simulink model "CAVE_MachE_driver_test"  (R2024a)
settings: configuration reference "ConfigSetDesktopFixedStep" (kept outside this file)
PreLoadFcn:
  | VSS_BICYCLE=Simulink.Variant('Dual=0');
  | VSS_DUAL=Simulink.Variant('Dual=1');
  | Dual=1;
  | load('DriveCycle2.mat')
PostLoadFcn:
  | if any(exist('dsrtsu_mdlpostloadfcn', 'file') ~= 0), dsrtsu_mdlpostloadfcn('Execute', bdroot); end
InitFcn:
  | , if any(exist('rtifpga_mdlclblib', 'file') ~= 0), rtifpga_mdlclblib('Init', bdroot); end,
  | , if any(exist('dsmpb_private', 'file') ~= 0), dsmpb_private('dsmpb_mdlclblib', 'Init', bdroot); end,
  | load('DriveCycle2.mat')
model workspace (MAT data in the model file):
  Gas = 0.383333333333
values from neighbouring files (symbols this model uses):
  CoastDown =     [Run_Simulink.mat]
  limitedMCT =     [Run_Simulink.mat]
  MCT =     [Run_Simulink.mat]
  optimized_speed = [6.8451519807e-19 6.71455685751e-19 6.61817305122e-19 6.79712455505e-19 6.66916107161e-19 6.93956205717e-19 6.71488581248e-19 6.61948887111e-19 6.81653289829e-19 6.68560882013e-19 6.9214695338e-19 6.73330729082e-19 ... (16417 elements, 16417x1)]    [OptimizedSpeed.mat]
  optimized_speed_time = [0 0.1 0.2 0.3 0.4 0.5 0.6 0.7 0.8 0.9 1 1.1 ... (16417 elements, 16417x1)]    [OptimizedSpeed.mat]
  pMCT =     [Run_Simulink.mat]
  RealSimPara =     [Run_Simulink.mat]
  Ref_speed = [13 13.007895099 13.015778396 13.023649891 13.031509584 13.039357475 13.047193564 13.055017851 13.062830336 13.070631019 13.0784199 13.086196979 ... (2669 elements, 2669x1)]    [Ref_speed_and_time.mat]
  Ref_time = [0 0.01 0.02 0.03 0.04 0.05 0.06 0.07 0.08 0.09 0.1 0.11 ... (2669 elements, 2669x1)]    [Ref_speed_and_time.mat]
  US06 =     [Run_Simulink.mat]
undefined symbols (not defined in the file or in its folder): AccelCmd, ActTqLF_Nm_, ActTqLR_Nm_, ActTqRF_Nm_, ActTqRR_Nm_, BattChargeLimitMaxPwr, BattChargeLimitSocBpts, BattChargeLimitTbl, BattChrgCapcty, BattDischargeLimitSocBpts, BattDischargeLimitTbl, BattDischargeMaxPwr, BattNumCellsParallel, BattNumCellsSeries, BattOpenVoltCapBpts, BattOpenVoltTbl, BattResistSocBpts, BattResistTbl, BattResistTempBpts, BrakeMaxPrs, BrakeMaxTrq, ChassisDistCg2FrontAxle, ChassisDistCg2RearAxle, ChassisVehMass, CltchCmd, DecelCmd, DiffRatio, DiscIntNeverNeededParam, EnvGravCnst, EnvPrs, EnvTemp, FuelSpecificGrav, GearCmd, h, InitStates, lgSw, MtrEffSpdBpts, MtrEffTbl, MtrEffTrqBpts, MtrPwrMax, MtrTrqMax, ResultsDrivingTests, SteeringCmd, SupvsryCtrlRegenBrkCutOffTbl, SupvsryCtrlRegenSpdBpts, TestScnrioCycleNum, VEH
libraries: simulink x122, VSIGenLib x122, etargetslib x75, dsmpblib x55, vehdynlibtire x24, autolibshared x22, CarMaker4SL x20, vehdynlibsuspension x14, vehdynlibtirecommon x14, autolibutils x10, VsrLibWheel x8, autolibpowerinfoutils x6
(part 12 of 32)

== system CAVE_MachE_driver_test/Vehicle Under Test3/Vehicle/Battery/Battery/Lithium Ion Battery Pack1 ==
  note: Info
  BattCurr : Inport  Unit=A
  BattTemp : Inport  Port=2  Unit=K
  Datasheet Battery Internal : Subsystem  AncestorBlock=autolibbatterycommon/Datasheet Battery Internal
  Info Bus : autolibbatterycommon/Info  RefBlkName='autolibdatasheetbattery/Datasheet Battery'
  Output Passthrough : autolibbatterycommon/Output Passthrough  SystemSampleTime=-1  VariantActivationTime=update diagram  AllowFlexibleInterface=on  Latency=0  AutoFrameSizeCalculation=off
  Info : Outport  VectorParamsAs1DForOutWhenUnconnected=off
  BattVolt : Outport  Port=2  Unit=V  VectorParamsAs1DForOutWhenUnconnected=off
  wires:
  [BattPwrLoss] -> Info Bus/5
  Output Passthrough/1 -> BattVolt/1, [BattVolt]
  [BattVolt] -> Info Bus/4
  Datasheet Battery Internal/1(LdCurrFeed) -> [LdCurrFeed]
  [LdCurrFeed] -> Info Bus/3
  Datasheet Battery Internal/5(BattPwrLoss) -> [BattPwrLoss]
  Datasheet Battery Internal/2(OutVoltUnfilt) -> Output Passthrough/1
  Datasheet Battery Internal/3(LdAmpHr) -> [LdAmpHr]
  Datasheet Battery Internal/4(BattSoc) -> [BattSoc]
  BattTemp/1 -> Datasheet Battery Internal/2(BattTemp)
  BattCurr/1 -> Datasheet Battery Internal/1(BattCurr)
  Info Bus/1 -> Info/1
  [BattSoc] -> Info Bus/2
  [LdAmpHr] -> Info Bus/1

== system CAVE_MachE_driver_test/Vehicle Under Test3/Vehicle/Driver and Drive Cycle/Driver and PI with FF Control/Speed controller set ==
  RefSpd [km/hr] : Inport
  VehSpd : Inport  Port=2
  Control selection : Constant
  In-house CAVE : Subsystem  VariantControl=varaint1
  Multiport Switch1 : MultiPortSwitch  SaturateOnIntegerOverflow=off  InputSameDT=off
  Multiport Switch2 : MultiPortSwitch  SaturateOnIntegerOverflow=off  InputSameDT=off
  Multiport Switch3 : MultiPortSwitch  SaturateOnIntegerOverflow=off  InputSameDT=off
  PIF : Subsystem  VariantControl=varaint2
  Predictive : Subsystem  VariantControl=varaint3
  Scope : Scope  NumInputPorts=2
  Speed tracking controller : Subsystem  Commented=on  Variant=on  VariantControlMode=label  VariantControl=Variant1  LabelModeActiveChoice=varaint1  PropagateVariantConditions=on
  Out1 : Outport
  Out2 : Outport  Port=2
  Out3 : Outport  Port=3
  wires:
  Control selection/1 -> Multiport Switch3/1, Multiport Switch2/1, Multiport Switch1/1
  RefSpd [km/hr]/1 -> Scope/1, In-house CAVE/1(RefSpd [km/hr]), Predictive/1(RefSpd [km/hr]), PIF/1(RefSpd [km/hr])
  In-house CAVE/1(AccelPedalCmd) -> Multiport Switch1/2
  PIF/1(AccelPedalCmd) -> Multiport Switch1/3
  Predictive/1(AccelPedalCmd) -> Multiport Switch1/4
  In-house CAVE/2(BrakePedalCmd) -> Multiport Switch2/2
  PIF/2(BrakePedalCmd) -> Multiport Switch2/3
  Predictive/2(BrakePedalCmd) -> Multiport Switch2/4
  In-house CAVE/3(Out3) -> Multiport Switch3/2
  PIF/3(Out3) -> Multiport Switch3/3
  Predictive/3(Out3) -> Multiport Switch3/4
  Multiport Switch3/1 -> Out3/1  "BrakeSwitch"
  Multiport Switch2/1 -> Out2/1  "BrakePedalCmd"
  Multiport Switch1/1 -> Out1/1  "AccelPedalCmd"
  VehSpd/1 -> Scope/2, In-house CAVE/2(In2), PIF/2(In2), Predictive/2(In2)

== system CAVE_MachE_driver_test/Vehicle Under Test3/Vehicle/Front Wheel Drive/Ideal Diff/Power Bus ==
  DriveshftTrq : Inport
  Speed : Inport  Port=2
  Bus Creator : BusCreator  Inputs=1
  Bus Creator5 : BusCreator  Inputs=2
  Bus Creator6 : BusCreator  Inputs=3
  Bus Creator7 : BusCreator  Inputs=1
  Constant : Constant  Value=0
  Constant1 : Constant  Value=0
  Constant2 : Constant  Value=0
  Demux : Demux  Outputs=3
  Power Accounting Bus Creator : autolibpowerinfoutils/Power Accounting Bus Creator  AssctBlkSelPopup=Parent reference block  RefBlkName='autolibshareddiff/Open Differential'  PwrTrnsfrdCheckBox=on  PwrNotTrnsfrdCheckBox=on  PwrStoredCheckBox=on  aMode=aMode
  Signal Specification5 : SignalSpecification  Unit=W
  Transferred Power : Product
  Vector Concatenate : Concatenate  NumInputs=3
  PwrInfo : Outport
  wires:
  Bus Creator/1 -> Power Accounting Bus Creator/1
  Power Accounting Bus Creator/1 -> PwrInfo/1  "PwrInfo"
  Bus Creator5/1 -> Power Accounting Bus Creator/2
  Bus Creator6/1 -> Bus Creator/1  "PwrTrnsfrd"
  Transferred Power/1 -> Signal Specification5/1
  Signal Specification5/1 -> Vector Concatenate/3, Vector Concatenate/2, Vector Concatenate/1  "PwrDriveshft"
  Constant/1 -> Bus Creator5/1  "PwrMechLoss"
  Demux/3 -> Bus Creator6/3  "PwrAxl2"
  DriveshftTrq/1 -> Transferred Power/1
  Bus Creator7/1 -> Power Accounting Bus Creator/3
  Demux/2 -> Bus Creator6/2  "PwrAxl1"
  Demux/1 -> Bus Creator6/1  "PwrDriveshft"
  Speed/1 -> Transferred Power/2
  Vector Concatenate/1 -> Demux/1
  Constant1/1 -> Bus Creator5/2  "PwrDampLoss"
  Constant2/1 -> Bus Creator7/1  "PwrStoredShft"

== system CAVE_MachE_driver_test/Vehicle Under Test3/Vehicle/Front Wheel Drive/Ideal Diff AWD/Power Bus ==
  DriveshftTrq : Inport
  Speed : Inport  Port=2
  Bus Creator : BusCreator  Inputs=1
  Bus Creator5 : BusCreator  Inputs=2
  Bus Creator6 : BusCreator  Inputs=3
  Bus Creator7 : BusCreator  Inputs=1
  Constant : Constant  Value=0
  Constant1 : Constant  Value=0
  Constant2 : Constant  Value=0
  Demux : Demux  Outputs=3
  Power Accounting Bus Creator : autolibpowerinfoutils/Power Accounting Bus Creator  AssctBlkSelPopup=Parent reference block  RefBlkName='autolibshareddiff/Open Differential'  PwrTrnsfrdCheckBox=on  PwrNotTrnsfrdCheckBox=on  PwrStoredCheckBox=on  aMode=aMode
  Signal Specification5 : SignalSpecification  Unit=W
  Transferred Power : Product
  Vector Concatenate : Concatenate  NumInputs=3
  PwrInfo : Outport
  wires:
  Bus Creator/1 -> Power Accounting Bus Creator/1
  Power Accounting Bus Creator/1 -> PwrInfo/1  "PwrInfo"
  Bus Creator5/1 -> Power Accounting Bus Creator/2
  Bus Creator6/1 -> Bus Creator/1  "PwrTrnsfrd"
  Transferred Power/1 -> Signal Specification5/1
  Signal Specification5/1 -> Vector Concatenate/3, Vector Concatenate/2, Vector Concatenate/1  "PwrDriveshft"
  Constant/1 -> Bus Creator5/1  "PwrMechLoss"
  Demux/3 -> Bus Creator6/3  "PwrAxl2"
  DriveshftTrq/1 -> Transferred Power/1
  Bus Creator7/1 -> Power Accounting Bus Creator/3
  Demux/2 -> Bus Creator6/2  "PwrAxl1"
  Demux/1 -> Bus Creator6/1  "PwrDriveshft"
  Speed/1 -> Transferred Power/2
  Vector Concatenate/1 -> Demux/1
  Constant1/1 -> Bus Creator5/2  "PwrDampLoss"
  Constant2/1 -> Bus Creator7/1  "PwrStoredShft"

== system CAVE_MachE_driver_test/Vehicle Under Test3/Vehicle/Front Wheel Drive/Real Diff/Power Bus ==
  DriveshftTrq : Inport
  Speed : Inport  Port=2
  Bus Creator : BusCreator  Inputs=1
  Bus Creator5 : BusCreator  Inputs=2
  Bus Creator6 : BusCreator  Inputs=3
  Bus Creator7 : BusCreator  Inputs=1
  Constant : Constant  Value=0
  Constant1 : Constant  Value=0
  Constant2 : Constant  Value=0
  Demux : Demux  Outputs=3
  Power Accounting Bus Creator : autolibpowerinfoutils/Power Accounting Bus Creator  AssctBlkSelPopup=Parent reference block  RefBlkName='autolibshareddiff/Open Differential'  PwrTrnsfrdCheckBox=on  PwrNotTrnsfrdCheckBox=on  PwrStoredCheckBox=on  aMode=aMode
  Signal Specification5 : SignalSpecification  Unit=W
  Transferred Power : Product
  Vector Concatenate : Concatenate  NumInputs=3
  PwrInfo : Outport
  wires:
  Bus Creator/1 -> Power Accounting Bus Creator/1
  Power Accounting Bus Creator/1 -> PwrInfo/1  "PwrInfo"
  Bus Creator5/1 -> Power Accounting Bus Creator/2
  Bus Creator6/1 -> Bus Creator/1  "PwrTrnsfrd"
  Transferred Power/1 -> Signal Specification5/1
  Signal Specification5/1 -> Vector Concatenate/3, Vector Concatenate/2, Vector Concatenate/1  "PwrDriveshft"
  Constant/1 -> Bus Creator5/1  "PwrMechLoss"
  Demux/3 -> Bus Creator6/3  "PwrAxl2"
  DriveshftTrq/1 -> Transferred Power/1
  Bus Creator7/1 -> Power Accounting Bus Creator/3
  Demux/2 -> Bus Creator6/2  "PwrAxl1"
  Demux/1 -> Bus Creator6/1  "PwrDriveshft"
  Speed/1 -> Transferred Power/2
  Vector Concatenate/1 -> Demux/1
  Constant1/1 -> Bus Creator5/2  "PwrDampLoss"
  Constant2/1 -> Bus Creator7/1  "PwrStoredShft"

== system CAVE_MachE_driver_test/Vehicle Under Test3/Vehicle/Powertrain Supervisory Controller /Engine Torque Command/Accel Pedal to Traction Wheel Torque Request1 ==
  note: Convert Accelerator Pedal Position to Torque Command
      | using Motor Torque Speed Curve
  AccelPdl : Inport
  MotSpd : Inport  Port=2
  Max Motor Torque : Subsystem
  Product1 : Product
  TrqCmd : Outport  VectorParamsAs1DForOutWhenUnconnected=off
  wires:
  Max Motor Torque/1(MtrTrqMax) -> Product1/2
  MotSpd/1 -> Max Motor Torque/1(MtrSpd)
  AccelPdl/1 -> Product1/1
  Product1/1 -> TrqCmd/1

== system CAVE_MachE_driver_test/Vehicle Under Test3/Vehicle/Powertrain Supervisory Controller /Engine Torque Command/Battery Management System ==
  note: Behaviorial BMS System. Limits battery charge / discharge power based on SOC.
      |
      | Charge/Discharge Limits and curves can be adjusted if using a larger battery pack
      | or motor power is changed.
  SOC : Inport
  ChrgLmt : Lookup_n-D  NumberOfTableDimensions=1  BreakpointsForDimension1=BattChargeLimitSocBpts  Table=BattChargeLimitTbl  ExtrapMethod=Clip  UseLastTableValue=on  InternalRulePriority=Speed  RndMeth=Simplest
  DischrgLmt : Lookup_n-D  NumberOfTableDimensions=1  BreakpointsForDimension1=BattDischargeLimitSocBpts  Table=BattDischargeLimitTbl  ExtrapMethod=Clip  UseLastTableValue=on  InternalRulePriority=Speed  RndMeth=Simplest
  MaxChrg : Constant  Value=BattChargeLimitMaxPwr
  MaxDischrg : Constant  Value=BattDischargeMaxPwr
  Product : Product
  Product1 : Product
  BattPwrDischrgLmt : Outport  VectorParamsAs1DForOutWhenUnconnected=off
  BattPwrChrgLmt : Outport  Port=2  VectorParamsAs1DForOutWhenUnconnected=off
  wires:
  DischrgLmt/1 -> Product/1
  ChrgLmt/1 -> Product1/1
  Product1/1 -> BattPwrChrgLmt/1
  Product/1 -> BattPwrDischrgLmt/1
  MaxDischrg/1 -> Product/2
  MaxChrg/1 -> Product1/2
  SOC/1 -> ChrgLmt/1, DischrgLmt/1

== system CAVE_MachE_driver_test/Vehicle Under Test3/Vehicle/Powertrain Supervisory Controller /Engine Torque Command/Motor Torque Arbitration and Power Management ==
  MotTrqCmdTrac : Inport
  AccelPdl : Inport  Port=2
  BattPwrDisChrgLmt : Inport  Port=3
  "BattPwrChrgLmt " : Inport  Port=4
  MotSpd : Inport  Port=5
  MotTrqCmdRegen : Inport  Port=6
  Accel Decel Switch : Switch  Criteria=u2 > Threshold  SaturateOnIntegerOverflow=off  InputSameDT=off
  Compare To Constant : simulink/Logic and Bit Operations/Compare To Constant  relop=>  const=0  OutDataTypeStr=boolean
  Power Management : Subsystem
  MotTrqCmdFinal : Outport  VectorParamsAs1DForOutWhenUnconnected=off
  wires:
  Compare To Constant/1 -> Accel Decel Switch/2
  MotSpd/1 -> Power Management/3(MotSpd)
  "BattPwrChrgLmt "/1 -> Power Management/2(BattPwrChrgLmt)
  BattPwrDisChrgLmt/1 -> Power Management/1(BattPwrDischrgLmt)
  Accel Decel Switch/1 -> Power Management/4(MotTrqCmd)
  Power Management/1(MotTrqCmdFinal) -> MotTrqCmdFinal/1
  MotTrqCmdTrac/1 -> Accel Decel Switch/1
  MotTrqCmdRegen/1 -> Accel Decel Switch/3
  AccelPdl/1 -> Compare To Constant/1

== system CAVE_MachE_driver_test/Vehicle Under Test3/Vehicle/Powertrain Supervisory Controller /Engine Torque Command/Series Regen Braking ==
  note: These are all torque on wheels, which is DiffRatio*torque on motor
  note: - Total brake torque request based on brake pressure and parameters of disc brakes
      | - Use as much regenerative motor braking as possible
      | - Any braking torque request that cannot be provided by the motor, will be provided by the friction brakes
  BattSoc : Inport
  VehSpd : Inport  Port=2
  MotSpd : Inport  Port=3
  "DecelCmd " : Inport  Port=4
  ChrgLmt : Lookup_n-D  NumberOfTableDimensions=1  BreakpointsForDimension1=BattChargeLimitSocBpts  Table=BattChargeLimitTbl  ExtrapMethod=Clip  UseLastTableValue=on  InternalRulePriority=Speed  RndMeth=Simplest
  Gain : Gain  Gain=-1
  Gain1 : Gain  Gain=BrakeMaxTrq
  Gain2 : Gain  Gain=1/BrakeMaxTrq
  Max Motor Torque : LibPtSupervisoryCtrl/Powertrain Supervisory Controller /Engine Torque Command/Accel Pedal to Traction Wheel Torque Request/Max Motor Torque  SystemSampleTime=-1  VariantActivationTime=update diagram  AllowFlexibleInterface=on  Latency=0  AutoFrameSizeCalculation=off
  MinMax : MinMax  Inputs=2
  MotTrqReflectedToWheels : Gain  Gain=DiffRatio
  Product1 : Product
  Product3 : Product
  RegenBrakingCutoff : Lookup_n-D  NumberOfTableDimensions=1  BreakpointsForDimension1=SupvsryCtrlRegenSpdBpts  Table=SupvsryCtrlRegenBrkCutOffTbl  ExtrapMethod=Clip  UseLastTableValue=on  InternalRulePriority=Speed  RndMeth=Simplest
  Saturation : Saturate  UpperLimit=1  LowerLimit=0
  Saturation1 : Saturate  UpperLimit=1  LowerLimit=0
  Subtract : Sum  Inputs=+-
  WhlTrqReflectedToMot : Gain  Gain=1/DiffRatio
  " MotTrqCmdRegen" : Outport  VectorParamsAs1DForOutWhenUnconnected=off
  " BrkCmd" : Outport  Port=2  VectorParamsAs1DForOutWhenUnconnected=off
  wires:
  Gain2/1 -> Saturation1/1  "BrkTrqReqTotal"
  Subtract/1 -> Gain2/1
  Saturation/1 -> Gain1/1
  "DecelCmd "/1 -> Saturation/1  "BrkPrsReq"
  Gain/1 -> " MotTrqCmdRegen"/1  "MotTrqCmdRegen"
  WhlTrqReflectedToMot/1 -> Gain/1
  MotTrqReflectedToWheels/1 -> MinMax/2  "MotTrqMaxWhls"
  MotSpd/1 -> Max Motor Torque/1
  BattSoc/1 -> ChrgLmt/1
  Product1/1 -> Product3/2  "RegenFactor"
  RegenBrakingCutoff/1 -> Product1/1
  VehSpd/1 -> RegenBrakingCutoff/1
  ChrgLmt/1 -> Product1/2
  MinMax/1 -> Product3/1  "min"
  Max Motor Torque/1 -> MotTrqReflectedToWheels/1  "MotTrqMax"
  Saturation1/1 -> " BrkCmd"/1
  Product3/1 -> Subtract/2, WhlTrqReflectedToMot/1  "MotTrqRegenWhl"
  Gain1/1 -> MinMax/1, Subtract/1  "BrkTrqReqTotal"

== system CAVE_MachE_driver_test/Vehicle Under Test3/Vehicle/Rototest and ORNL Interface/From Rototest/RotoTestEthRX ==
  Input : Inport
  Depacker : Subsystem
  Floater{,1..15} (16 alike) : VSIGenLib/Floater  SystemSampleTime=-1  VariantActivationTime=update diagram  AllowFlexibleInterface=on  Latency=0  AutoFrameSizeCalculation=off
  Header : VSIGenLib/Header  not=''
  Selector1 : Selector  IndexMode=Zero-based  InputPortWidth=96  IndexOptions=Index vector (dialog)  Indices=[3 2]  OutputSizes=1
  Selector10 : Selector  IndexMode=Zero-based  InputPortWidth=96  IndexOptions=Index vector (dialog)  Indices=[35 34 33 32]  OutputSizes=1
  Selector11 : Selector  IndexMode=Zero-based  InputPortWidth=96  IndexOptions=Index vector (dialog)  Indices=[39 38 37 36]  OutputSizes=1
  Selector12 : Selector  IndexMode=Zero-based  InputPortWidth=96  IndexOptions=Index vector (dialog)  Indices=[43 42 41 40]  OutputSizes=1
  Selector13 : Selector  IndexMode=Zero-based  InputPortWidth=96  IndexOptions=Index vector (dialog)  Indices=[47 46 45 44]  OutputSizes=1
  Selector14 : Selector  IndexMode=Zero-based  InputPortWidth=96  IndexOptions=Index vector (dialog)  Indices=[51 50 49 48]  OutputSizes=1
  Selector15 : Selector  IndexMode=Zero-based  InputPortWidth=96  IndexOptions=Index vector (dialog)  Indices=[55 54 53 52]  OutputSizes=1
  Selector16 : Selector  IndexMode=Zero-based  InputPortWidth=96  IndexOptions=Index vector (dialog)  Indices=[59 58 57 56]  OutputSizes=1
  Selector17 : Selector  IndexMode=Zero-based  InputPortWidth=96  IndexOptions=Index vector (dialog)  Indices=[63 62 61 60]  OutputSizes=1
  Selector18 : Selector  IndexMode=Zero-based  InputPortWidth=96  IndexOptions=Index vector (dialog)  Indices=[67 66 65 64]  OutputSizes=1
  Selector19 : Selector  IndexMode=Zero-based  InputPortWidth=96  IndexOptions=Index vector (dialog)  Indices=[71 70 69 68]  OutputSizes=1
  Selector2 : Selector  IndexMode=Zero-based  InputPortWidth=96  IndexOptions=Index vector (dialog)  Indices=[7 6 5 4]  OutputSizes=1
  Selector20 : Selector  IndexMode=Zero-based  InputPortWidth=96  IndexOptions=Index vector (dialog)  Indices=[75 74 73 72]  OutputSizes=1
  Selector21 : Selector  IndexMode=Zero-based  InputPortWidth=96  IndexOptions=Index vector (dialog)  Indices=[79 78 77 76]  OutputSizes=1
  Selector22 : Selector  IndexMode=Zero-based  InputPortWidth=96  IndexOptions=Index vector (dialog)  Indices=[83 82 81 80]  OutputSizes=1
  Selector23 : Selector  IndexMode=Zero-based  InputPortWidth=96  IndexOptions=Index vector (dialog)  Indices=[85 84]  OutputSizes=1
  Selector24 : Selector  IndexMode=Zero-based  InputPortWidth=96  IndexOptions=Index vector (dialog)  Indices=[87 86]  OutputSizes=1
  Selector25 : Selector  IndexMode=Zero-based  InputPortWidth=96  IndexOptions=Index vector (dialog)  Indices=[89 88]  OutputSizes=1
  Selector26 : Selector  IndexMode=Zero-based  InputPortWidth=96  IndexOptions=Index vector (dialog)  Indices=[91 90]  OutputSizes=1
  Selector27 : Selector  IndexMode=Zero-based  InputPortWidth=96  IndexOptions=Index vector (dialog)  Indices=[93 92]  OutputSizes=1
  Selector28 : Selector  IndexMode=Zero-based  InputPortWidth=96  IndexOptions=Index vector (dialog)  Indices=[94]  OutputSizes=1
  Selector29 : Selector  IndexMode=Zero-based  InputPortWidth=96  IndexOptions=Index vector (dialog)  Indices=[95]  OutputSizes=1
  Selector3 : Selector  IndexMode=Zero-based  InputPortWidth=96  IndexOptions=Index vector (dialog)  Indices=[1 0]  OutputSizes=1
  Selector4 : Selector  IndexMode=Zero-based  InputPortWidth=96  IndexOptions=Index vector (dialog)  Indices=[11 10 9 8]  OutputSizes=1
  Selector5 : Selector  IndexMode=Zero-based  InputPortWidth=96  IndexOptions=Index vector (dialog)  Indices=[15 14 13 12]  OutputSizes=1
  Selector6 : Selector  IndexMode=Zero-based  InputPortWidth=96  IndexOptions=Index vector (dialog)  Indices=[19 18 17 16]  OutputSizes=1
  Selector7 : Selector  IndexMode=Zero-based  InputPortWidth=96  IndexOptions=Index vector (dialog)  Indices=[23 22 21 20]  OutputSizes=1
  Selector8 : Selector  IndexMode=Zero-based  InputPortWidth=96  IndexOptions=Index vector (dialog)  Indices=[27 26 25 24]  OutputSizes=1
  Selector9 : Selector  IndexMode=Zero-based  InputPortWidth=96  IndexOptions=Index vector (dialog)  Indices=[31 30 29 28]  OutputSizes=1
  Terminator{,1..2,7..8} (5 alike) : Terminator
  uint16 (unsigned 16){1..7} (7 alike) : etargetslib/Byte Unpack  dimensions={[1]}  datatypes={'uint16'}  byteAlign=1
  uint32 (unsigned 32){1..4} (4 alike) : etargetslib/Byte Unpack  dimensions={[1]}  datatypes={'uint32'}  byteAlign=1
  uint8 (unsigned 8)1 : etargetslib/Byte Unpack  dimensions={[1]}  datatypes={'uint8'}  byteAlign=1
  uint8 (unsigned 8)2 : etargetslib/Byte Unpack  dimensions={[1]}  datatypes={'uint8'}  byteAlign=1
  ID : Outport
  ProtocolVer : Outport  Port=2
  ActTqLF_Nm : Outport  Port=3
  ActSpLF_rpm : Outport  Port=4
  ActTempLF_C : Outport  Port=5
  ActTqRF_Nm_ : Outport  Port=6
  ActSpRF_rpm : Outport  Port=7
  ActTempRF_C : Outport  Port=8
  ActTqLR_Nm : Outport  Port=9
  ActSpLR_rpm : Outport  Port=10
  ActTempLR_C : Outport  Port=11
  ActTqRR_Nm : Outport  Port=12
  ActSpRR_rpm : Outport  Port=13
  ActTempRR_Nm : Outport  Port=14
  RefLF_Nm : Outport  Port=15
  RefRF_rpm : Outport  Port=16
  RefLR_Nm : Outport  Port=17
  RefRR_Nm : Outport  Port=18
  UnitsStatusLF : Outport  Port=19
  UnitsStatusRF : Outport  Port=20
  UnitsStatusLR : Outport  Port=21
  UnitsStatusRR : Outport  Port=22
  WatchdogCnt : Outport  Port=23
  FaultActive : Outport  Port=24
  WarningsActive : Outport  Port=25
  SpTqRR : Outport  Port=26
  SpTqLR : Outport  Port=27
  SpTqRF : Outport  Port=28
  SpTqLF : Outport  Port=29
  SystemActive : Outport  Port=30
  wires:
  Depacker/7(SystemActive) -> SystemActive/1
  Depacker/5(SpTqRF) -> SpTqRF/1
  Depacker/1(FaultActive) -> FaultActive/1
  Depacker/2(WarningsActive) -> WarningsActive/1
  Depacker/3(SpTqRR) -> SpTqRR/1
  Depacker/4(SpTqLR) -> SpTqLR/1
  Depacker/6(SpTqLF) -> SpTqLF/1
  Floater5/1 -> ActTempRF_C/1  "ActTempRF_C"
  uint32 (unsigned 32)2/1 -> Terminator1/1  "Reserved"
  Floater/1 -> ActSpLF_rpm/1  "ActSpLF_rpm"
  uint32 (unsigned 32)1/1 -> Terminator/1  "Reserved"
  uint16 (unsigned 16)1/1 -> ID/1  "ID"
  Floater15/1 -> RefRR_Nm/1  "RefRR_Nm"
  uint8 (unsigned 8)1/1 -> WatchdogCnt/1  "WatchdogCnt"
  Floater14/1 -> RefRF_rpm/1  "RefRF_rpm"
  uint16 (unsigned 16)5/1 -> UnitsStatusRF/1  "UnitsStatusRF"
  uint32 (unsigned 32)3/1 -> Terminator2/1  "Reserved"
  Floater9/1 -> ActSpRR_rpm/1  "ActSpRR_rpm"
  Floater1/1 -> ActTqLF_Nm/1  "ActTqLF_Nm_"
  Floater2/1 -> ActTempLF_C/1  "ActTempLF_C"
  Floater12/1 -> RefLF_Nm/1  "RefLF_Nm"
  Floater7/1 -> ActTqLR_Nm/1  "ActTqLR_Nm_"
  uint16 (unsigned 16)2/1 -> ProtocolVer/1  "ProtocolVer"
  Selector24/1 -> uint16 (unsigned 16)4/1
  Selector7/1 -> Floater4/1
  Selector8/1 -> Floater3/1
  uint16 (unsigned 16)7/1 -> UnitsStatusRR/1  "UnitsStatusRR"
  Selector22/1 -> Floater15/1
  Selector18/1 -> uint32 (unsigned 32)4/1
  Selector12/1 -> Floater6/1
  Selector23/1 -> uint16 (unsigned 16)3/1
  uint16 (unsigned 16)6/1 -> UnitsStatusLR/1  "UnitsStatusLR"
  Selector17/1 -> Floater11/1
  uint16 (unsigned 16)4/1 -> UnitsStatusLF/1  "UnitsStatusLF"
  Selector27/1 -> uint16 (unsigned 16)7/1
  Floater13/1 -> RefLR_Nm/1  "RefLR_Nm"
  Selector14/1 -> uint32 (unsigned 32)3/1
  Selector2/1 -> Floater1/1
  Selector13/1 -> Floater8/1
  Selector26/1 -> uint16 (unsigned 16)6/1
  Selector6/1 -> uint32 (unsigned 32)1/1
  uint16 (unsigned 16)3/1 -> Depacker/1(SysStsBits)  "SystemStatusBits"
  uint32 (unsigned 32)4/1 -> Terminator7/1  "Reserved"
  Floater3/1 -> ActSpRF_rpm/1  "ActSpRF_rpm"
  Selector25/1 -> uint16 (unsigned 16)5/1
  Floater4/1 -> ActTqRF_Nm_/1  "ActTqRF_Nm_"
  uint8 (unsigned 8)2/1 -> Terminator8/1  "Reserved"
  Floater11/1 -> ActTempRR_Nm/1  "ActTempRR_Nm"
  Floater6/1 -> ActSpLR_rpm/1  "ActSpLR_rpm"
  Selector20/1 -> Floater14/1
  Selector9/1 -> Floater5/1
  Selector5/1 -> Floater2/1
  Selector15/1 -> Floater10/1
  Selector16/1 -> Floater9/1
  Floater8/1 -> ActTempLR_C/1  "ActTempLR_C"
  Selector3/1 -> uint16 (unsigned 16)1/1
  Selector28/1 -> uint8 (unsigned 8)1/1
  Selector29/1 -> uint8 (unsigned 8)2/1
  Selector21/1 -> Floater13/1
  Input/1 -> Selector7/1, Selector8/1, Selector9/1, Selector10/1, Selector11/1, Selector12/1, Selector13/1, Selector17/1, Selector18/1, Selector19/1, Selector20/1, Selector21/1, Selector22/1, Selector23/1, Selector25/1, Selector26/1, Selector27/1, Selector29/1, Selector28/1, Selector24/1, Selector16/1, Selector15/1, Selector14/1, Selector6/1, Selector5/1, Selector4/1, Selector2/1, Selector1/1, Selector3/1
  Selector19/1 -> Floater12/1
  Selector10/1 -> uint32 (unsigned 32)2/1
  Selector1/1 -> uint16 (unsigned 16)2/1
  Selector4/1 -> Floater/1
  Floater10/1 -> ActTqRR_Nm/1  "ActTqRR_Nm_"
  Selector11/1 -> Floater7/1

== system CAVE_MachE_driver_test/Vehicle Under Test3/Vehicle/Rototest and ORNL Interface/Get Wheel Spd Cmd Based on Wheel Dynamics/WheelSpdCmd ==
  In1 : Inport
  Bus Selector : BusSelector  OutputSignals=PT IF WFL rotv,PT IF WFR rotv,PT IF WRL rotv,PT IF WRR rotv
  Mux : Mux
  Out1 : Outport
  wires:
  Mux/1 -> Out1/1
  Bus Selector/1 -> Mux/1  "<PT IF WFL rotv>"
  Bus Selector/4 -> Mux/4  "<PT IF WRR rotv>"
  In1/1 -> Bus Selector/1
  Bus Selector/3 -> Mux/3  "<PT IF WRL rotv>"
  Bus Selector/2 -> Mux/2  "<PT IF WFR rotv>"

== system CAVE_MachE_driver_test/Vehicle Under Test3/Vehicle/Rototest and ORNL Interface/Get Wheel Spd Cmd Based on Wheel Dynamics/Whl Dynamics & Format CM Powertrain Signal ==
  note: include regen!!
  note: Based on tire model
  note: Can Bypass with my own brake model
  BrakingTorques : Inport
  Trq_T2W : Inport  Port=2
  AxlTrq : Inport  Port=3
  MaxRegen : Inport  Port=4
  FxIn : Inport  Port=5
  Bus Creator2 : BusCreator  Inputs=42
  Bus Selector : BusSelector  OutputSignals=Car Trq_T2WFL,Car Trq_T2WFR,Car Trq_T2WRL,Car Trq_T2WRR
  Bus Selector2 : BusSelector  OutputSignals=Brake IF Trq_WB FL,Brake IF Trq_WB FR,Brake IF Trq_WB RL,Brake IF Trq_WB RR
  BusCreator1 : BusCreator  Inputs=42
  Constant : Constant  Value=500
  Demux : Demux
  Demux1 : Demux
  Demux2 : Demux  Outputs=42
      settings: DisplayOption=none
  Diff Trq : Subsystem
  Discrete-Time Integrator{4..7} (4 alike) : DiscreteIntegrator  IntegratorMethod=Integration: Backward Euler  SampleTime=-1  ICPrevOutput=DiscIntNeverNeededParam  ICPrevScaledInput=DiscIntNeverNeededParam
  Gain{5..8} (4 alike) : Gain  Gain=-1
  Ground{2..5} (4 alike) : Ground
  Ignition : Constant
  Memory{1..4} (4 alike) : Memory
  Operation Error : Constant  Value=4
  Operation State Driving : Constant  Value=4
  Product{1..4} (4 alike) : Product  RndMeth=Zero
  Saturation{1..4} (4 alike) : Saturate  UpperLimit=1  LowerLimit=-1
  Subsystem : Subsystem
  Subsystem1 : Subsystem  Commented=on
  Subsystem2 : Subsystem
  Subsystem3 : Subsystem
  Subsystem4 : Subsystem
  Subsystem5 : Subsystem  Commented=on
  Subsystem6 : Subsystem  Commented=on
  Subsystem7 : Subsystem  Commented=on
  Zero{1..5} (5 alike) : Constant  Value=0
  PowerTrainOutIdeal : Outport
  tag scope: AxlTqrRotoTest=global
  wires:
  Saturation4/1 -> Product4/2
  Memory4/1 -> Saturation4/1
  Bus Selector2/4 -> Product4/1  "<Brake IF Trq_WB RR>"
  Product4/1 -> Subsystem4/1(BrakeTorq), Gain8/1  "BrakeTrqRR"
  Saturation2/1 -> Product2/2
  Memory2/1 -> Saturation2/1
  Bus Selector2/3 -> Product2/1  "<Brake IF Trq_WB RL>"
  Product2/1 -> Subsystem3/1(BrakeTorq), Gain7/1  "BrakeTrqRL"
  Saturation1/1 -> Product1/2
  Memory1/1 -> Saturation1/1
  Bus Selector2/2 -> Product1/1  "<Brake IF Trq_WB FR>"
  Product1/1 -> Subsystem2/1(BrakeTorq), Gain6/1  "BrakeTrqFR"
  Memory3/1 -> Saturation3/1
  Saturation3/1 -> Product3/2
  Bus Selector2/1 -> Product3/1  "<Brake IF Trq_WB FL>"
  Product3/1 -> Subsystem/1(BrakeTorq), Gain5/1  "BrakeTrqFL"
  BrakingTorques/1 -> Bus Selector2/1
  Trq_T2W/1 -> Bus Selector/1
  Discrete-Time Integrator7/1 -> Bus Creator2/36  "PtT WRR rot"
  Discrete-Time Integrator6/1 -> Bus Creator2/29  "PT WRL rot"
  Discrete-Time Integrator5/1 -> Bus Creator2/22  "PT WFR rot"
  Discrete-Time Integrator4/1 -> Bus Creator2/15  "PT WFL rot"
  Ignition/1 -> Bus Creator2/1  "PT Ignition"
  Bus Creator2/1 -> Demux2/1
  Operation State Driving/1 -> Bus Creator2/2
  Operation Error/1 -> Bus Creator2/3
  Zero1/1 -> Bus Creator2/5, Bus Creator2/4, Bus Creator2/12, Bus Creator2/14, Bus Creator2/13, Bus Creator2/11, Bus Creator2/10, Bus Creator2/9, Bus Creator2/8
  Zero2/1 -> Bus Creator2/19, Bus Creator2/20
  Zero3/1 -> Bus Creator2/26, Bus Creator2/27
  Zero4/1 -> Bus Creator2/32, Bus Creator2/33, Bus Creator2/34, Bus Creator2/35
  Zero5/1 -> Bus Creator2/39, Bus Creator2/40, Bus Creator2/41, Bus Creator2/42
  Gain6/1 -> Bus Creator2/24
  Gain5/1 -> Bus Creator2/17
  Gain7/1 -> Bus Creator2/31
  Gain8/1 -> Bus Creator2/38
  Demux2/42 -> BusCreator1/42  "PT IF WRR Trq_BrakeReg_max"
  Demux2/41 -> BusCreator1/41  "PT IF WRR Trq_BrakeReg"
  Demux2/40 -> BusCreator1/40  "PT IF WRR Trq_Supp2WC"
  Demux2/39 -> BusCreator1/39  "PT IF WRR Trq_Drive"
  Demux2/38 -> BusCreator1/38  "PT IF WRR Trq_B2W"
  Demux2/37 -> BusCreator1/37  "PT IF WRR rotv"
  Demux2/36 -> BusCreator1/36  "PT IF WRR rot"
  Demux2/35 -> BusCreator1/35  "PT IF WRL Trq_BrakeReg_max"
  Demux2/34 -> BusCreator1/34  "PT IF WRL Trq_BrakeReg"
  Demux2/33 -> BusCreator1/33  "PT IF WRL Trq_Supp2WC"
  Demux2/32 -> BusCreator1/32  "PT IF WRL Trq_Drive"
  Demux2/31 -> BusCreator1/31  "PT IF WRL Trq_B2W"
  Demux2/30 -> BusCreator1/30  "PT IF WRL rotv"
  Demux2/29 -> BusCreator1/29  "PT IF WRL rot"
  Demux2/28 -> BusCreator1/28  "PT IF WFR Trq_BrakeReg_max"
  Demux2/27 -> BusCreator1/27  "PT IF WFR Trq_BrakeReg"
  Demux2/26 -> BusCreator1/26  "PT IF WFR Trq_Supp2WC"
  Demux2/25 -> BusCreator1/25  "PT IF WFR Trq_Drive"
  Demux2/24 -> BusCreator1/24  "PT IF WFR Trq_B2W"
  Demux2/23 -> BusCreator1/23  "PT IF WFR rotv"
  Demux2/22 -> BusCreator1/22  "PT IF WFR rot"
  Demux2/21 -> BusCreator1/21  "PT IF WFL Trq_BrakeReg_max"
  Demux2/20 -> BusCreator1/20  "PT IF WFL Trq_BrakeReg"
  Demux2/19 -> BusCreator1/19  "PT IF WFL Trq_Supp2WC"
  Demux2/18 -> BusCreator1/18  "PT IF WFL Trq_Drive"
  Demux2/17 -> BusCreator1/17  "PT IF WFL Trq_B2W"
  Demux2/16 -> BusCreator1/16  "PT IF WFL rotv"
  Demux2/15 -> BusCreator1/15  "PT IF WFL rot"
  Demux2/14 -> BusCreator1/14  "PT IF DL_iDiff_mean"
  Demux2/13 -> BusCreator1/13  "PT IF Trq_Supp2BdyEng y"
  Demux2/12 -> BusCreator1/12  "PT IF Trq_Supp2BdyEng x"
  Demux2/11 -> BusCreator1/11  "PT IF Trq_Supp2Bdy1B z"
  Demux2/10 -> BusCreator1/10  "PT IF Trq_Supp2Bdy1B y"
  Demux2/9 -> BusCreator1/9  "PT IF Trq_Supp2Bdy1B x"
  Demux2/8 -> BusCreator1/8  "PT IF Trq_Supp2Bdy1 z"
  Demux2/7 -> BusCreator1/7  "PT IF Trq_Supp2Bdy1 y"
  Demux2/6 -> BusCreator1/6  "PT IF Trq_Supp2Bdy1 x"
  Demux2/5 -> BusCreator1/5  "PT IF Engine_rotv"
  Demux2/4 -> BusCreator1/4  "PT IF GearNo"
  Demux2/3 -> BusCreator1/3  "PT IF OperationError"
  Demux2/2 -> BusCreator1/2  "PT IF OperationState"
  Demux2/1 -> BusCreator1/1  "PT IF Ignition"
  BusCreator1/1 -> PowerTrainOutIdeal/1
  Ground2/1 -> Bus Creator2/7
  Ground4/1 -> Bus Creator2/6
  Constant/1 -> Diff Trq/1(In1)
  AxlTrq/1 -> [AxlTqrRotoTest], Demux/1
  Demux/1 -> Subsystem/3(AxlTorq), Bus Creator2/25, Bus Creator2/18
  MaxRegen/1 -> Bus Creator2/28, Bus Creator2/21
  Subsystem/1(rotv FL) -> Subsystem3/5(FWSpd), Subsystem4/5(FWSpd), Bus Creator2/16, Memory3/1, Discrete-Time Integrator4/1
  Bus Selector/1 -> Subsystem/2(<Car Trq_T2WFL>)  "<Car Trq_T2WFL>"
  Subsystem2/1(rotv FR) -> Bus Creator2/23, Memory1/1, Discrete-Time Integrator5/1
  Bus Selector/2 -> Subsystem2/2(<Car Trq_T2WFR>)  "<Car Trq_T2WFR>"
  Demux/2 -> Subsystem2/3(AxlTorq)
  Subsystem3/1(rotv RL) -> Memory2/1, Discrete-Time Integrator6/1, Bus Creator2/30
  Bus Selector/3 -> Subsystem3/2(<Car Trq_T2WRL>)  "<Car Trq_T2WRL>"
  Demux/3 -> Subsystem3/3(AxlTorq)
  Subsystem4/1(rotv RR) -> Memory4/1, Discrete-Time Integrator7/1, Bus Creator2/37
  Bus Selector/4 -> Subsystem4/2(<Car Trq_T2WRR>)  "<Car Trq_T2WRR>"
  Demux/4 -> Subsystem4/3(AxlTorq)
  FxIn/1 -> Demux1/1
  Demux1/1 -> Subsystem/4(Fx)
  Demux1/2 -> Subsystem2/4(Fx)
  Demux1/3 -> Subsystem3/4(Fx)
  Demux1/4 -> Subsystem4/4(Fx)

== system CAVE_MachE_driver_test/Vehicle Under Test3/Vehicle/Rototest and ORNL Interface/To Rototest with Band-Aid/Band-Aid ==
  InSpd_rpm : Inport
  InTrq_Nm : Inport  Port=2
  BRAKE_PRESSED : Inport  Port=3
  VehSpd_kph : Inport  Port=4
  Band-Aid : Stateflow chart  TreatAsAtomicUnit=on
  BrkLatchThr_Nm : Constant  Value=-50
  Header : VSIGenLib/Header  not=''
  LaunchSpdThr_rpm : Constant  Value=2
  LaunchTrqThr_Nm : Constant  Value=20
  SettleTime_s : Constant  Value=5
  SpdLatchThr_rpm : Constant  Value=1e-5
  Terminator : Terminator
  Terminator1 : Terminator
  VehSpdThr_kph : Constant  Value=0.2
  dStop : Constant  Value=0
  OutMode : Outport
  OutSpd_rpm : Outport  Port=2
  tag scope: Mode=global
  wires:
  InSpd_rpm/1 -> Band-Aid/5(InSpd)  "InSpd_rpm"
  LaunchTrqThr_Nm/1 -> Band-Aid/2(LaunchTrqThr)
  SpdLatchThr_rpm/1 -> Band-Aid/3(SpdLatchThr)
  Band-Aid/3(State) -> Terminator/1  "State"
  LaunchSpdThr_rpm/1 -> Band-Aid/1(LaunchSpdThr)
  SettleTime_s/1 -> Band-Aid/7(SettleTime)
  Band-Aid/1(OutMode) -> [Mode], OutMode/1  "OutMode"
  BrkLatchThr_Nm/1 -> Terminator1/1
  Band-Aid/2(OutSpd) -> OutSpd_rpm/1  "OutSpd"
  InTrq_Nm/1 -> Band-Aid/6(InTrq)  "InTrq_Nm"
  dStop/1 -> Band-Aid/8(dStop)
  BRAKE_PRESSED/1 -> Band-Aid/4(BrkSw)
  VehSpd_kph/1 -> Band-Aid/9(VehSpd_kph)  "VehicleSpeed_kph"
  VehSpdThr_kph/1 -> Band-Aid/10(VehSpdThr_kph)

== system CAVE_MachE_driver_test/Vehicle Under Test3/Vehicle/Rototest and ORNL Interface/To Rototest with Band-Aid/Logging ==
  Ground1 : Ground
  RotoTestEthRXLogging : Subsystem
      mask Display:
      | color('white')
      | disp('RotTestEthLog')
      | port_label('output', 1, 'ID')
      | port_label('output', 2, 'ProtocolVer')
      | port_label('output', 3, 'ActTqLF (Nm)')
      | port_label('output', 4, 'ActSpdLF (rpm)')
      | port_label('output', 5, 'ActTempLF (C)')
      | port_label('output', 6, 'ActTqRF (Nm)')
      | port_label('output', 7, 'ActSpRF (rpm)')
      | port_label('output', 8, 'ActTempRF (C)')
      | port_label('output', 9, 'ActTqLR (Nm)')
      | port_label('output', 10, 'ActSpLR (rpm)')
      | port_label('output', 11, 'ActTempLR (C)')
      | port_label('output', 12, 'ActTqRR (Nm)')
      | port_label('output', 13, 'ActSpRR (rpm)')
      | port_label('output', 14, 'ActTempRR (Nm)')
      | port_label('output', 15, 'ActTqDeltaF (Nm)')
      | port_label('output', 16, 'ActSpDeltaF (rpm)')
      | port_label('output', 17, 'ActTqDeltaR (Nm)')
      | port_label('output', 18, 'ActSpDeltaR (rpm)')
      | port_label('output', 19, 'ActTqDeltaA (Nm')
      | port_label('output', 20, 'ActSqDeltaA (rpm)')
      | port_label('output', 21, 'ActTqTot (Nm)')
      | port_label('output', 22, 'ActSpAve (rpm)')
      | port_label('output', 23, 'ActPow (kW)')
      | port_label('output', 24, 'ActVehSp (kph)')
      | port_label('output', 25, 'TPTime (ms)')
      | port_label('output', 26, 'TPDistance (m)')
      | port_label('output', 27, 'FaultActive (bool)')
      | port_label('output', 28, 'WarningsActive (bool)')
      | port_label('output', 29, 'MeasuringStatus (bool)')
      | port_label('output', 30, 'SystemActive (bool)')
      | 
      | port_label('output', 31, 'UnitStatusLF (enum)')
      | port_label('output', 32, 'UnitStatusRF (enum)')
      | port_label('output', 33, 'UnitStatusLR (enum)')
      | port_label('output', 34, 'UnitStatusRR (enum)')
      | port_label('output', 35, 'WatchdogCnt (int)')
  Terminator{28..62} (35 alike) : Terminator
  wires:
  RotoTestEthRXLogging/24(ActVehSp_kph) -> Terminator51/1
  RotoTestEthRXLogging/9(ActTqLR_Nm) -> Terminator30/1
  RotoTestEthRXLogging/11(ActTempLR_C) -> Terminator38/1
  RotoTestEthRXLogging/5(ActTempLF_C) -> Terminator28/1
  RotoTestEthRXLogging/12(ActTqRR_Nm) -> Terminator39/1
  RotoTestEthRXLogging/10(ActSpLR_rpm) -> Terminator31/1
  RotoTestEthRXLogging/8(ActTempRF_C) -> Terminator33/1
  RotoTestEthRXLogging/26(TPDistance_m) -> Terminator59/1
  RotoTestEthRXLogging/19(ActTqDeltaA_Nm) -> Terminator44/1
  RotoTestEthRXLogging/6(ActTqRF_Nm) -> Terminator29/1
  RotoTestEthRXLogging/4(ActSpLF_rpm) -> Terminator37/1
  RotoTestEthRXLogging/1(ID) -> Terminator34/1
  RotoTestEthRXLogging/14(ActTempRR_Nm) -> Terminator47/1
  RotoTestEthRXLogging/30(SystemActive) -> Terminator53/1
  RotoTestEthRXLogging/22(ActSpAve_rpm) -> Terminator43/1
  RotoTestEthRXLogging/13(ActSpRR_rpm) -> Terminator46/1
  RotoTestEthRXLogging/31(UnitsStatusLF) -> Terminator56/1
  RotoTestEthRXLogging/21(ActTqTot_Nm) -> Terminator42/1
  RotoTestEthRXLogging/17(ActTqDeltaR_Nm) -> Terminator40/1
  RotoTestEthRXLogging/7(ActSpRF_rpm) -> Terminator32/1
  RotoTestEthRXLogging/2(ProtocolVer) -> Terminator35/1
  RotoTestEthRXLogging/16(ActSpDeltaF_rpm) -> Terminator49/1
  RotoTestEthRXLogging/18(ActSpDeltaR_rpm) -> Terminator41/1
  RotoTestEthRXLogging/15(ActTqDeltaF_Nm) -> Terminator48/1
  RotoTestEthRXLogging/33(UnitsStatusLR) -> Terminator54/1
  RotoTestEthRXLogging/23(ActPow_kW) -> Terminator50/1
  RotoTestEthRXLogging/25(TPTime_ms) -> Terminator58/1
  RotoTestEthRXLogging/28(WarningsActive) -> Terminator61/1
  RotoTestEthRXLogging/27(FaultActive) -> Terminator60/1
  RotoTestEthRXLogging/35(WatchdogCnt) -> Terminator62/1
  RotoTestEthRXLogging/34(UnitsStatusRR) -> Terminator55/1
  RotoTestEthRXLogging/20(ActSpDeltaA_rpm) -> Terminator45/1
  RotoTestEthRXLogging/32(UnitsStatusRF) -> Terminator57/1
  RotoTestEthRXLogging/29(MeasuringStatus) -> Terminator52/1
  RotoTestEthRXLogging/3(ActTqLF_Nm) -> Terminator36/1
  Ground1/1 -> RotoTestEthRXLogging/1(Cmd)

== system CAVE_MachE_driver_test/Vehicle Under Test3/Vehicle/Rototest and ORNL Interface/To Rototest with Band-Aid/Mode Override ==
  Header : VSIGenLib/Header  not=''
  Mux6 : Mux
  SpTqLF : Constant  Value=0  OutDataTypeStr=uint8
  SpTqLR : Constant  Value=0  OutDataTypeStr=uint8
  SpTqRF : Constant  Value=0  OutDataTypeStr=uint8
  SpTqRR : Constant  Value=0  OutDataTypeStr=uint8
  Ovr : Outport
  wires:
  Mux6/1 -> Ovr/1
  SpTqRR/1 -> Mux6/1
  SpTqLR/1 -> Mux6/2
  SpTqRF/1 -> Mux6/3
  SpTqLF/1 -> Mux6/4

== system CAVE_MachE_driver_test/Vehicle Under Test3/Vehicle/Rototest and ORNL Interface/To Rototest with Band-Aid/RotoTestEthTx ==
  RefLF_NmORrpm : Inport
  RefRF_NmORrpm : Inport  Port=2
  RefLR_NmORrpm : Inport  Port=3
  RefRR_NmORrpm : Inport  Port=4
  SpTqRR : Inport  Port=5
  SpTqLR : Inport  Port=6
  SpTqRF : Inport  Port=7
  SpTqLF : Inport  Port=8
  SystemActive : Inport  Port=9
  Constant : Constant  Value=255  OutDataTypeStr=uint8
  Constant1 : Constant  Value=0  OutDataTypeStr=uint8
  Constant2 : Constant  Value=0  OutDataTypeStr=uint8
  Constant3 : Constant  Value=0  OutDataTypeStr=uint8
  Defloater{,1..3} (4 alike) : VSIGenLib/Defloater  SystemSampleTime=-1  VariantActivationTime=update diagram  AllowFlexibleInterface=on  Latency=0  AutoFrameSizeCalculation=off
  Demux{,1..3} (4 alike) : Demux
  Header : VSIGenLib/Header  not=''
  ID1 : Constant  Value=hex2dec('D3')  OutDataTypeStr=uint8
  ID2 : Constant  Value=hex2dec('02')  OutDataTypeStr=uint8
  MATLAB Function : MATLAB Function  TreatAsAtomicUnit=on
  Mux : Mux  Inputs=25
  Packer : Subsystem
  ProtocolVer : Constant  Value=0  OutDataTypeStr=uint16
  SystemCtrlBits2 : Constant  Value=0  OutDataTypeStr=uint8
  Terminator : Terminator
  WatchdogCnt : simulink/Sources/Counter Free-Running  NumBits=8  tsamp=-1
  uint16 (unsigned 16) 2 : etargetslib/Byte Pack  datatypes={'uint16'}  byteAlign=1
  uint8 (unsigned 8) {1..9} (9 alike) : etargetslib/Byte Pack  datatypes={'uint8'}  byteAlign=1
  Output : Outport
  wires:
  Defloater2/1 -> Demux2/1
  ID2/1 -> uint8 (unsigned 8) 7/1
  RefRF_NmORrpm/1 -> Defloater1/1  "RefRF_NmORrpm"
  Demux1/4 -> Mux/11
  Constant1/1 -> uint8 (unsigned 8) 4/1  "Reserved25"
  WatchdogCnt/1 -> uint8 (unsigned 8) 1/1  "WatchdogCnt"
  Defloater3/1 -> Demux3/1
  Demux3/3 -> Mux/18
  uint8 (unsigned 8) 5/1 -> Mux/21
  Demux1/3 -> Mux/10
  uint8 (unsigned 8) 2/1 -> Mux/23
  Constant2/1 -> uint8 (unsigned 8) 3/1  "Reserved24"
  ID1/1 -> uint8 (unsigned 8) 8/1
  uint8 (unsigned 8) 4/1 -> Mux/25
  Demux/1 -> Mux/4
  Demux3/1 -> Mux/16
  Demux1/1 -> Mux/8
  ProtocolVer/1 -> uint16 (unsigned 16) 2/1
  uint8 (unsigned 8) 3/1 -> Mux/24
  Demux2/2 -> Mux/13
  uint8 (unsigned 8) 1/1 -> Mux/22
  uint16 (unsigned 16) 2/1 -> Mux/3
  Defloater1/1 -> Demux1/1
  Defloater/1 -> Demux/1
  Demux2/1 -> Mux/12
  Demux/4 -> Mux/7
  Demux2/3 -> Mux/14
  MATLAB Function/1(y) -> uint8 (unsigned 8) 9/1  "Ref_Byte"
  Demux1/2 -> Mux/9
  Demux/3 -> Mux/6
  Mux/1 -> Output/1  "bytesend"
  uint8 (unsigned 8) 8/1 -> Mux/1
  Demux2/4 -> Mux/15
  Demux3/4 -> Mux/19
  SystemCtrlBits2/1 -> uint8 (unsigned 8) 5/1  "SystemCtrlBits2"
  uint8 (unsigned 8) 7/1 -> Mux/2
  RefRR_NmORrpm/1 -> Defloater3/1  "RefRR_NmORrpm"
  Demux/2 -> Mux/5
  Constant3/1 -> uint8 (unsigned 8) 2/1  "Reserved23"
  Demux3/2 -> Mux/17
  RefLF_NmORrpm/1 -> Defloater/1  "RefLF_NmORrpm"
  RefLR_NmORrpm/1 -> Defloater2/1  "RefLR_NmORrpm"
  SpTqRR/1 -> MATLAB Function/1(SpTqRR), Packer/1(SpTqRR)  "SpTqRR"
  SpTqLR/1 -> MATLAB Function/2(SpTqLR), Packer/2(SpTqLR)  "SpTqLR"
  SpTqRF/1 -> MATLAB Function/3(SpTqRF), Packer/3(SpTqRF)  "SpTqRF"
  SpTqLF/1 -> MATLAB Function/4(SpTqLF), Packer/4(SpTqLF)  "SpTqLF"
  SystemActive/1 -> MATLAB Function/5(SystemActive), Packer/5(SystemActive)
  Packer/1(SystemCtrlBits) -> Terminator/1
  Constant/1 -> uint8 (unsigned 8) 6/1
  uint8 (unsigned 8) 9/1 -> Mux/20

== system CAVE_MachE_driver_test/Vehicle Under Test3/Vehicle/Rototest and ORNL Interface/To Rototest with Band-Aid/TrqSpd Override ==
  Header : VSIGenLib/Header  not=''
  Mux2 : Mux
  RefLF_NmORrpm : Constant  Value=0
  RefLR_NmORrpm : Constant  Value=0
  RefRF_NmORrpm : Constant  Value=0
  RefRR_NmORrpm : Constant  Value=0
  Ovr : Outport
  wires:
  RefRF_NmORrpm/1 -> Mux2/2
  RefLF_NmORrpm/1 -> Mux2/1
  RefLR_NmORrpm/1 -> Mux2/3
  RefRR_NmORrpm/1 -> Mux2/4
  Mux2/1 -> Ovr/1

== system CAVE_MachE_driver_test/Vehicle Under Test3/Vehicle/Vehicle Dynamics/Vehicle 14DOF/Brake Pressure ==
  BrkReq : Inport
  Bus Creator1 : BusCreator  Inputs=2
  Gain : Gain  Gain=BrakeMaxPrs
  Gain{1..4} (4 alike) : Gain  Gain=0.5
  Saturation{,1..3} (4 alike) : Saturate  UpperLimit=BrakeMaxPrs  LowerLimit=0  ZeroCross=off
  Signal Specification : SignalSpecification  Unit=Pa
  Terminator : Terminator
  Vector Concatenate2 : Concatenate  NumInputs=4
  BrakePrs : Outport  Unit=Pa
  wires:
  BrkReq/1 -> Gain/1, Bus Creator1/1  "BrkReq"
  Gain/1 -> Signal Specification/1
  Signal Specification/1 -> Gain2/1, Gain1/1, Bus Creator1/2  "BrkPrs"
  Bus Creator1/1 -> Terminator/1  "WhlBrk"
  Gain1/1 -> Gain4/1
  Gain2/1 -> Gain3/1
  Gain3/1 -> Saturation/1, Saturation1/1
  Gain4/1 -> Saturation2/1, Saturation3/1
  Vector Concatenate2/1 -> BrakePrs/1
  Saturation/1 -> Vector Concatenate2/1
  Saturation1/1 -> Vector Concatenate2/2
  Saturation2/1 -> Vector Concatenate2/3
  Saturation3/1 -> Vector Concatenate2/4

== system CAVE_MachE_driver_test/Vehicle Under Test3/Vehicle/Vehicle Dynamics/Vehicle 14DOF/Steering ==
  SteeringCmd : Inport
  Constant : Constant  Value=0
  Kinematic Steering : vehdynlibsteering/Kinematic Steering  StrgType=Parallel  StrgRatioType=Constant  Loc=Front  NrmlFctr=1  TrckWdth=1.9  WhlBase=ChassisDistCg2FrontAxle+ChassisDistCg2RearAxle  Db=0  StrgRng=2.91*pi  StrgAngBpts="[-6.2832   -5.0265   -3.7699   -2.5133   -1.2566         0    1.2566    2.5133    3.7699    5.0265    6.2832]"  StrgRatioTbl=|  StrgRatio=16.8  PctAckIn=off  PctAck=100  PctAckTbl=ones(1,11)*100  StrgArmLngth=0.1  RckCsLngth=0.5  TieRodLngth=0.248  D=0.2  PnnRadius=0.0057  PnnRadiusTbl="[0.0055    0.0055    0.0056    0.0057    0.0058    0.0057    0.0057    0.0057    0.0056    0.0055    0.0055]"  RodLngth=0.1  ParaArmLngth=0.9  aMode=2
      | [13.5000   13.3750   13.2500   13.1250   13.0000   13.0000   13.0000   13.1250   13.2500   13.3750   13.5000
      | ]
  Terminator1 : Terminator
  Vector Concatenate : Concatenate
  Vector Concatenate1 : Concatenate
  Vector Concatenate2 : Concatenate
  WhlAng : Outport  Unit=rad
  wires:
  Kinematic Steering/1 -> Terminator1/1
  Vector Concatenate2/1 -> WhlAng/1
  Kinematic Steering/2 -> Vector Concatenate/1
  Vector Concatenate1/1 -> Vector Concatenate2/2  "RearWheelAngles"
  Vector Concatenate/1 -> Vector Concatenate2/1  "FrontWheelAngles"
  Constant/1 -> Vector Concatenate1/2, Vector Concatenate1/1
  Kinematic Steering/3 -> Vector Concatenate/2
  SteeringCmd/1 -> Kinematic Steering/1

== system CAVE_MachE_driver_test/Vehicle Under Test3/Vehicle/Vehicle Dynamics/Vehicle 14DOF/Subsystem1 ==
  Cgxyzdot : Inport
  CgXYZ : Inport  Port=2
  CgXYZdot : Inport  Port=3
  angles : Inport  Port=4
  pqr : Inport  Port=5
  Cgaxyz : Inport  Port=6
  Beta : Inport  Port=7
  GeomXYZ : Inport  Port=8
  GeomXYZdot : Inport  Port=9
  Cgxyzdotdot : Inport  Port=10
  Omega : Inport  Port=11
  Kappa : Inport  Port=12
  Alpha : Inport  Port=13
  XWheel : Inport  Port=14
  YWheel : Inport  Port=15
  dzWheel : Inport  Port=16
  Bus Creator1 : BusCreator  Inputs=29
  Bus Creator3 : BusCreator  Inputs=6
  Demux{,1..8} (9 alike) : Demux  Outputs=3
  Scope : Scope
  Subsystem : Subsystem
  Chassis : Outport  VectorParamsAs1DForOutWhenUnconnected=off
  Wheels : Outport  Port=2  VectorParamsAs1DForOutWhenUnconnected=off
  wires:
  Demux8/3 -> Bus Creator1/3  "zdotdot"
  Demux8/2 -> Bus Creator1/2  "ydotdot"
  Demux8/1 -> Bus Creator1/1  "xdotdot"
  Cgxyzdotdot/1 -> Demux8/1
  Subsystem/1(VehSpd) -> Scope/1, Bus Creator1/29  "VehSpd"
  Demux7/3 -> Bus Creator1/28  "GeomZdot"
  Demux7/2 -> Bus Creator1/27  "GeomYdot"
  Demux7/1 -> Bus Creator1/26  "GeomXdot"
  Demux6/3 -> Bus Creator1/25  "GeomZ"
  Demux6/2 -> Bus Creator1/24  "GeomY"
  Demux6/1 -> Bus Creator1/23  "GeomX"
  Beta/1 -> Bus Creator1/22  "Beta"
  Demux5/3 -> Bus Creator1/21  "az"
  Demux5/2 -> Bus Creator1/20  "ay"
  Demux5/1 -> Bus Creator1/19  "ax"
  Demux4/3 -> Bus Creator1/18  "r"
  Demux4/2 -> Bus Creator1/17  "q"
  Demux4/1 -> Bus Creator1/16  "p"
  Demux3/3 -> Bus Creator1/15  "psi"
  Demux3/2 -> Bus Creator1/14  "theta"
  Demux3/1 -> Bus Creator1/13  "phi"
  Demux2/3 -> Bus Creator1/12  "Zdot"
  Demux2/2 -> Bus Creator1/11  "Ydot"
  Demux2/1 -> Bus Creator1/10  "Xdot"
  Demux1/3 -> Bus Creator1/9  "Z"
  Demux1/2 -> Bus Creator1/8  "Y"
  Demux1/1 -> Bus Creator1/7  "X"
  Demux/3 -> Bus Creator1/6  "zdot"
  Demux/2 -> Bus Creator1/5  "ydot"
  Demux/1 -> Bus Creator1/4  "xdot"
  GeomXYZ/1 -> Demux6/1
  GeomXYZdot/1 -> Demux7/1
  Cgaxyz/1 -> Demux5/1
  pqr/1 -> Demux4/1
  angles/1 -> Demux3/1, Subsystem/2(angles)
  CgXYZdot/1 -> Demux2/1
  CgXYZ/1 -> Demux1/1
  Cgxyzdot/1 -> Demux/1, Subsystem/1(Cgxyzdot)
  Alpha/1 -> Bus Creator3/2  "Alpha"
  XWheel/1 -> Bus Creator3/4  "XWheel"
  YWheel/1 -> Bus Creator3/5  "YWheel"
  Bus Creator3/1 -> Wheels/1  "Wheels"
  Kappa/1 -> Bus Creator3/1  "Kappa"
  dzWheel/1 -> Bus Creator3/6  "dZWheel"
  Omega/1 -> Bus Creator3/3  "Omega"
  Bus Creator1/1 -> Chassis/1  "Chassis"

== system CAVE_MachE_driver_test/Vehicle Under Test3/Vehicle/Vehicle Dynamics/Vehicle 14DOF/Subsystem4 ==
  Cgxyzdot : Inport
  CgXYZ : Inport  Port=2
  CgXYZdot : Inport  Port=3
  angles : Inport  Port=4
  pqr : Inport  Port=5
  Cgaxyz : Inport  Port=6
  Beta : Inport  Port=7
  GeomXYZ : Inport  Port=8
  GeomXYZdot : Inport  Port=9
  Omega : Inport  Port=10
  Kappa : Inport  Port=11
  Alpha : Inport  Port=12
  XWheel : Inport  Port=13
  YWheel : Inport  Port=14
  dzWheel : Inport  Port=15
  Bus Creator : BusCreator  Inputs=26
  Bus Creator3 : BusCreator  Inputs=6
  Demux{,1..7} (8 alike) : Demux  Outputs=3
  Subsystem : Subsystem
  Chassis : Outport  VectorParamsAs1DForOutWhenUnconnected=off
  Wheels : Outport  Port=2  VectorParamsAs1DForOutWhenUnconnected=off
  wires:
  Bus Creator/1 -> Chassis/1  "Chassis"
  Omega/1 -> Bus Creator3/3  "Omega"
  dzWheel/1 -> Bus Creator3/6  "dZWheel"
  Kappa/1 -> Bus Creator3/1  "Kappa"
  Bus Creator3/1 -> Wheels/1  "Wheels"
  YWheel/1 -> Bus Creator3/5  "YWheel"
  XWheel/1 -> Bus Creator3/4  "XWheel"
  Alpha/1 -> Bus Creator3/2  "Alpha"
  Cgxyzdot/1 -> Subsystem/1(Cgxyzdot), Demux/1
  CgXYZ/1 -> Demux1/1
  CgXYZdot/1 -> Demux2/1
  angles/1 -> Subsystem/2(angles), Demux3/1
  pqr/1 -> Demux4/1
  Cgaxyz/1 -> Demux5/1
  GeomXYZdot/1 -> Demux7/1
  GeomXYZ/1 -> Demux6/1
  Demux/1 -> Bus Creator/1  "xdot"
  Demux/2 -> Bus Creator/2  "ydot"
  Demux/3 -> Bus Creator/3  "zdot"
  Demux1/1 -> Bus Creator/4  "X"
  Demux1/2 -> Bus Creator/5  "Y"
  Demux1/3 -> Bus Creator/6  "Z"
  Demux2/1 -> Bus Creator/7  "Xdot"
  Demux2/2 -> Bus Creator/8  "Ydot"
  Demux2/3 -> Bus Creator/9  "Zdot"
  Demux3/1 -> Bus Creator/10  "phi"
  Demux3/2 -> Bus Creator/11  "theta"
  Demux3/3 -> Bus Creator/12  "psi"
  Demux4/1 -> Bus Creator/13  "p"
  Demux4/2 -> Bus Creator/14  "q"
  Demux4/3 -> Bus Creator/15  "r"
  Demux5/1 -> Bus Creator/16  "ax"
  Demux5/2 -> Bus Creator/17  "ay"
  Demux5/3 -> Bus Creator/18  "az"
  Beta/1 -> Bus Creator/19  "Beta"
  Demux6/1 -> Bus Creator/20  "GeomX"
  Demux6/2 -> Bus Creator/21  "GeomY"
  Demux6/3 -> Bus Creator/22  "GeomZ"
  Demux7/1 -> Bus Creator/23  "GeomXdot"
  Demux7/2 -> Bus Creator/24  "GeomYdot"
  Demux7/3 -> Bus Creator/25  "GeomZdot"
  Subsystem/1(VehSpd) -> Bus Creator/26  "VehSpd"
